simulink model "Aeropendulum_new_model"  (R2021b)
settings: Solver=VariableStepAuto  StartTime=0.0  StopTime=80.0  FixedStep=0.1  RelTol=1e-3
values from neighbouring files (symbols this model uses):
  c = 0.007    [ANM_params.m]    (also in ANM_params_test.m)
  d = 0.25    [ANM_params.m]    (also in ANM_params_test.m)
  g = 9.81    [ANM_params.m]    (also in ANM_params_test.m)
  J = m*l*l    (= 0.0075)    [ANM_params.m]    (also in ANM_params_test.m)
  l = 0.25    [ANM_params.m]    (also in ANM_params_test.m)
  m = 0.120    (= 0.12)    [ANM_params.m]    (also in ANM_params_test.m)
libraries: rllib x1, simulink x1
settings Model: Creator=Marcin  LastModifiedBy=Marcin

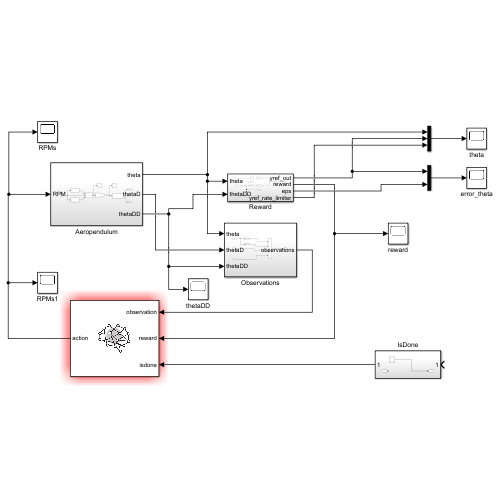
[thumbnail: Simulink's stored preview of the top-level diagram]
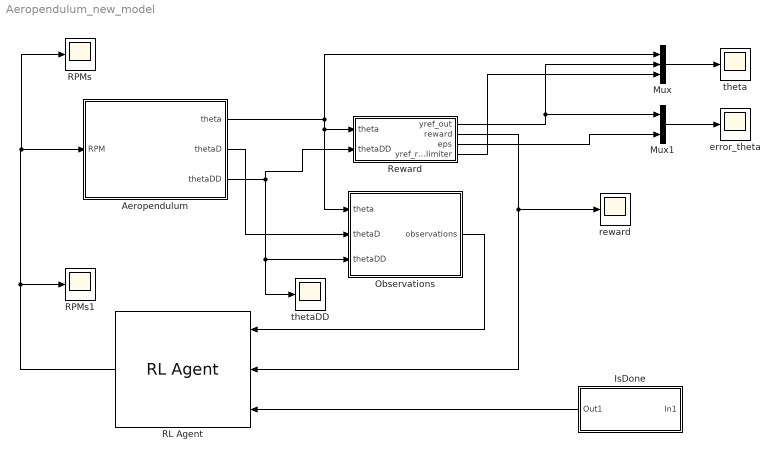
== system Aeropendulum_new_model ==
  Aeropendulum : Subsystem
  IsDone : Subsystem
  Mux : Mux  Inputs=3
  Mux1 : Mux  Inputs=2
  Observations : Subsystem
  RL Agent : rllib/RL Agent  Agent=agent  ExternalActionAsInput=off  ProvideCumRwd=off  TreatAsDirectFeedthrough=on
  RPMs : Scope
  RPMs1 : Scope
  Reward : Subsystem
  error_theta : Scope
  reward : Scope
  theta : Scope
  thetaDD : Scope
  wires:
  Reward/1(yref_out) -> Mux1/1, Mux/2
  Reward/2(reward) -> reward/1, RL Agent/2
  Observations/1(observations) -> RL Agent/1
  Mux/1 -> theta/1
  IsDone/1(Out1) -> RL Agent/3
  Mux1/1 -> error_theta/1
  Reward/3(eps) -> Mux1/2
  Aeropendulum/1(theta) -> Mux/1, Observations/1(theta), Reward/1(theta)
  Aeropendulum/2(thetaD) -> Observations/2(thetaD)
  Aeropendulum/3(thetaDD) -> Observations/3(thetaDD), thetaDD/1, Reward/2(thetaDD)
  RL Agent/1 -> RPMs/1, Aeropendulum/1(RPM), RPMs1/1
  Reward/4(yref_rate_limiter) -> Mux/3

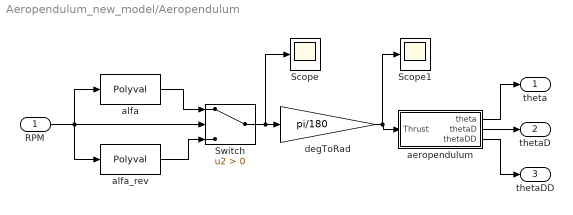
== system Aeropendulum_new_model/Aeropendulum ==
  RPM : Inport
  Scope : Scope
  Scope1 : Scope
  Switch : Switch  Criteria=u2 > Threshold
  aeropendulum : Subsystem
  alfa : Polyval  Coefs="[3.04986021927422e-06,  -0.00476887717971010 , 2.51670431281220]"
  alfa_rev : Polyval  Coefs="[-5.46944010985214e-06,\t-0.00938361577873603,\t-2.43262552689868]"
  degToRad : Gain  Gain=pi/180
  theta : Outport
  thetaD : Outport  Port=2
  thetaDD : Outport  Port=3
  wires:
  alfa/1 -> Switch/1
  RPM/1 -> alfa_rev/1, alfa/1, Switch/2
  Switch/1 -> Scope/1, degToRad/1
  degToRad/1 -> Scope1/1, aeropendulum/1(Thrust)
  alfa_rev/1 -> Switch/3
  aeropendulum/1(theta) -> theta/1
  aeropendulum/2(thetaD) -> thetaD/1
  aeropendulum/3(thetaDD) -> thetaDD/1

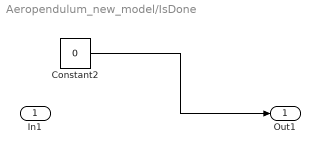
== system Aeropendulum_new_model/IsDone ==
  In1 : Inport
  Constant2 : Constant  Value=0
  Out1 : Outport
  wires:
  Constant2/1 -> Out1/1

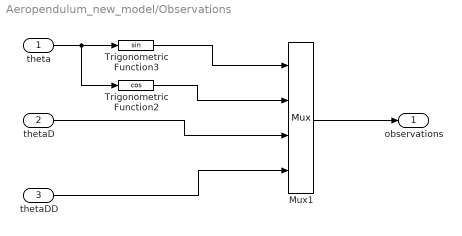
== system Aeropendulum_new_model/Observations ==
  theta : Inport
  thetaD : Inport  Port=2
  thetaDD : Inport  Port=3
  Mux1 : Mux
  Trigonometric Function2 : Trigonometry  Operator=cos
  Trigonometric Function3 : Trigonometry
  observations : Outport
  wires:
  Trigonometric Function3/1 -> Mux1/1
  theta/1 -> Trigonometric Function2/1, Trigonometric Function3/1
  Trigonometric Function2/1 -> Mux1/2
  Mux1/1 -> observations/1
  thetaD/1 -> Mux1/3
  thetaDD/1 -> Mux1/4

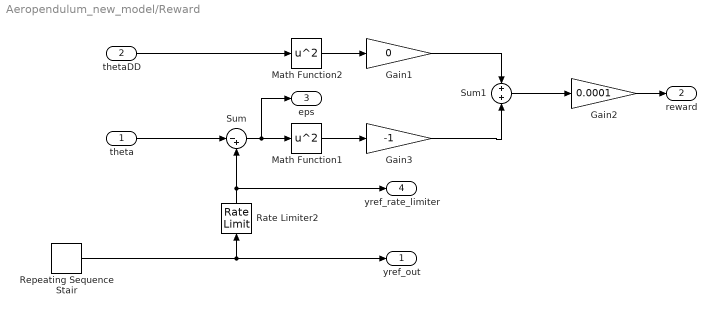
== system Aeropendulum_new_model/Reward ==
  theta : Inport
  thetaDD : Inport  Port=2
  Gain1 : Gain  Gain=0
  Gain2 : Gain  Gain=0.0001
  Gain3 : Gain  Gain=-1
  Math Function1 : Math  Operator=square  SignedPower=on  SaturateOnIntegerOverflow=on
  Math Function2 : Math  Operator=square  SignedPower=on  SaturateOnIntegerOverflow=on
  Rate Limiter2 : RateLimiter  SampleTimeMode=inherited
  Repeating Sequence Stair : simulink/Sources/Repeating Sequence Stair  OutValues=[10 20 30 40 50 60 70 80].'  tsamp=10  OutMin=[]  OutMax=[]  OutDataTypeStr=double  OutputDataTypeScalingMode=double  OutDataType=fixdt(0,8)  ConRadixGroup=Best Precision: Vector-wise  OutScaling=2^-12
  Sum : Sum  Inputs=|-+
  Sum1 : Sum
  yref_out : Outport
  reward : Outport  Port=2
  eps : Outport  Port=3
  yref_rate_limiter : Outport  Port=4
  wires:
  theta/1 -> Sum/1
  Sum/1 -> Math Function1/1, eps/1
  Gain3/1 -> Sum1/2
  thetaDD/1 -> Math Function2/1
  Math Function2/1 -> Gain1/1
  Gain1/1 -> Sum1/1
  Gain2/1 -> reward/1
  Sum1/1 -> Gain2/1
  Math Function1/1 -> Gain3/1
  Repeating Sequence Stair/1 -> Rate Limiter2/1, yref_out/1
  Rate Limiter2/1 -> yref_rate_limiter/1, Sum/2

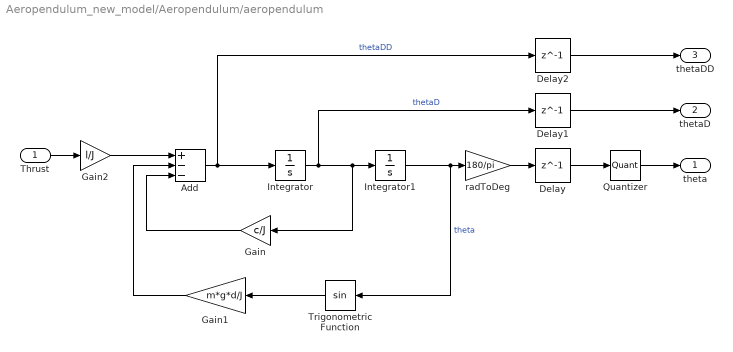
== system Aeropendulum_new_model/Aeropendulum/aeropendulum ==
  Thrust : Inport
  Add : Sum  Inputs=+--
  Delay : Delay  DelayLength=1  InitialCondition=0
  Delay1 : Delay  DelayLength=1  InitialCondition=0
  Delay2 : Delay  DelayLength=1  InitialCondition=0
  Gain : Gain  Gain=c/J
  Gain1 : Gain  Gain=m*g*d/J
  Gain2 : Gain  Gain=l/J
  Integrator : Integrator
  Integrator1 : Integrator
  Quantizer : Quantizer  QuantizationInterval=0.08791209
  Trigonometric Function : Trigonometry
  radToDeg : Gain  Gain=180/pi
  theta : Outport
  thetaD : Outport  Port=2
  thetaDD : Outport  Port=3
  wires:
  Thrust/1 -> Gain2/1
  Integrator/1 -> Delay1/1, Gain/1, Integrator1/1  "thetaD"
  Integrator1/1 -> Trigonometric Function/1, radToDeg/1  "theta"
  Add/1 -> Delay2/1, Integrator/1  "thetaDD"
  Gain1/1 -> Add/2
  Trigonometric Function/1 -> Gain1/1
  Gain/1 -> Add/3
  Gain2/1 -> Add/1
  radToDeg/1 -> Delay/1
  Delay1/1 -> thetaD/1
  Delay2/1 -> thetaDD/1
  Delay/1 -> Quantizer/1
  Quantizer/1 -> theta/1
